simulink model "Drive_Mode_Prueba (1)"  (R2025b)
settings: Solver=VariableStepAuto  StartTime=0.0  StopTime=10.0  RelTol=1e-3
libraries: Drive_Mode_Librery x1

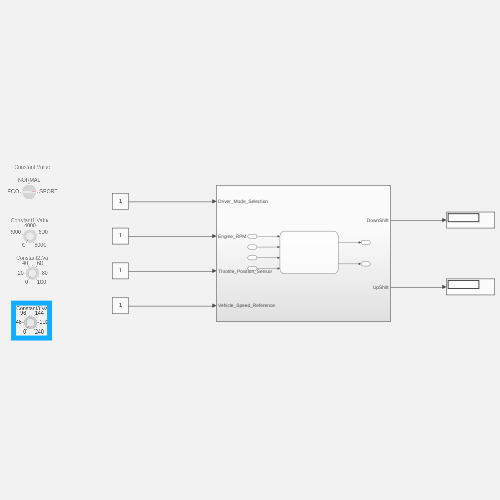
[thumbnail: Simulink's stored preview of the top-level diagram]
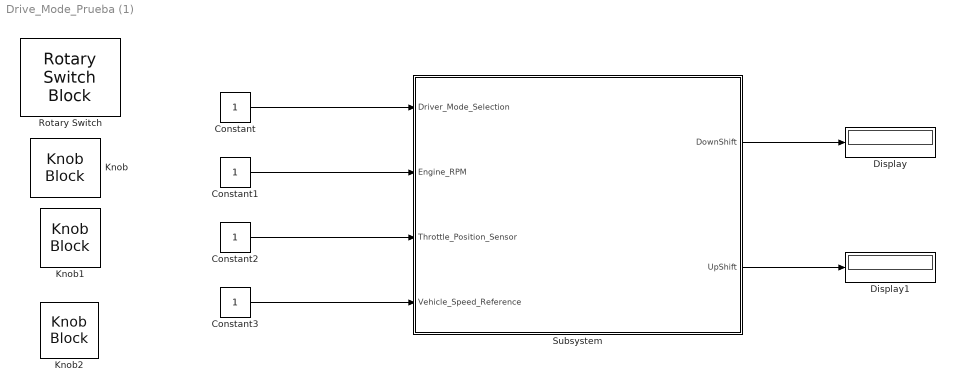
== system Drive_Mode_Prueba (1) ==
  Constant{,1..3} (4 alike) : Constant
  Display : Display
  Display1 : Display
  Knob : KnobBlock  ScaleMax=8000
  Knob1 : KnobBlock
  Knob2 : KnobBlock  ScaleMax=240
  Rotary Switch : RotarySwitchBlock
  Subsystem : Subsystem
  wires:
  Subsystem/1(DownShift) -> Display/1
  Subsystem/2(UpShift) -> Display1/1
  Constant3/1 -> Subsystem/4(Vehicle_Speed_Reference)
  Constant2/1 -> Subsystem/3(Throttle_Position_Sensor)
  Constant1/1 -> Subsystem/2(Engine_RPM)
  Constant/1 -> Subsystem/1(Driver_Mode_Selection)

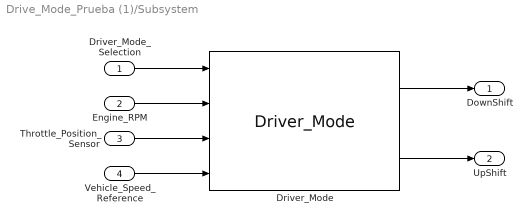
== system Drive_Mode_Prueba (1)/Subsystem ==
  Driver_Mode_Selection : Inport
  Engine_RPM : Inport  Port=2
  Throttle_Position_Sensor : Inport  Port=3
  Vehicle_Speed_Reference : Inport  Port=4
  Driver_Mode : Drive_Mode_Librery/Driver_Mode  SystemSampleTime=-1  VariantActivationTime=update diagram  EmptyChoice=off  PassThrough=off  PassThroughVariantControl=(default)  EmptyChoiceVariantControl=(default)  AllowFlexibleInterface=on  Latency=0  AutoFrameSizeCalculation=off
  DownShift : Outport
  UpShift : Outport  Port=2
  wires:
  Vehicle_Speed_Reference/1 -> Driver_Mode/4
  Throttle_Position_Sensor/1 -> Driver_Mode/3
  Engine_RPM/1 -> Driver_Mode/2
  Driver_Mode_Selection/1 -> Driver_Mode/1
  Driver_Mode/1 -> DownShift/1
  Driver_Mode/2 -> UpShift/1
